simulink model "Xe_Model_Redo_June_26"  (R2018a)
settings: Solver=VariableStepAuto  StartTime=0.0  StopTime=5E5+96*60*60  RelTol=1e-3
values from neighbouring files (symbols this model uses):
  A_pipe = pi*r_pipe^2    (= 0.0126676869774)    [Startup_Script.m]
  alpha_FS = 0.517E-16    (= 5.17e-17)    [Startup_Script.m]
  alpha_G_R1 = 0.334E-17    (= 3.34e-18)    [Startup_Script.m]
  alpha_G_R2 = 0.699E-17    (= 6.99e-18)    [Startup_Script.m]
  alpha_G_R3 = 0.669E-17    (= 6.69e-18)    [Startup_Script.m]
  alpha_G_R4 = 0.791E-18    (= 7.91e-19)    [Startup_Script.m]
  D_g = 2.37E-9    (= 2.37e-09)    [Startup_Script.m]
  epsilon = 0.1    [Startup_Script.m]
  eta_b = 1E-4    (= 0.0001)    [Startup_Script.m]
  eta_fs = 1.2E-4    (= 0.00012)    [Startup_Script.m]
  f_cv = 0.004    [Startup_Script.m]
  FS_Mu_A = 4340    [Startup_Script.m]
  FS_Mu_K = 0.084    [Startup_Script.m]
  FS_Mu_MSRE = 0.007027    [Startup_Script.m]
  FS_rho_A = 3.628    [Startup_Script.m]
  FS_rho_B = 0.00066    [Startup_Script.m]
  FS_rho_MSRE = 2082    [Startup_Script.m]
  gamma_i = 0.0293524    [Startup_Script.m]
  gamma_te = 0.0322482    [Startup_Script.m]
  gamma_xe = 0.00257324    [Startup_Script.m]
  h_fc = 1.6    [Startup_Script.m]
  H_Xe_a = 5.713e-13    [Startup_Script.m]
  H_Xe_b = -7.937e-10    [Startup_Script.m]
  H_Xe_c = 2.809e-07    [Startup_Script.m]
  HX_r_Tube = ((0.5-0.042)/2)*2.54E-2    (= 0.0058166)    [Startup_Script.m]
  HX_XS = HX_N_Tubes*(pi*HX_r_Tube^2)    (= 0.0168999490356)    [Startup_Script.m]
  k_b = 1.3806E-23    (= 1.3806e-23)    [Startup_Script.m]
  lambda_i = 2.9306070546251702E-5    (= 2.93060705463e-05)    [Startup_Script.m]
  lambda_te = 0.036481430555786593    (= 0.0364814305558)    [Startup_Script.m]
  lambda_xe = 2.0924e-05    [Startup_Script.m]
  N_FC_R1 = 12    [Startup_Script.m]
  N_FC_R2 = 940    [Startup_Script.m]
  N_FC_R3 = 108    [Startup_Script.m]
  N_FC_R4 = 78    [Startup_Script.m]
  P_pump = 35420    [Startup_Script.m]
  phi0 = 3.98E+17    (= 3.98e+17)    [Startup_Script.m]
  phi_G_R_1 = mean(interp1(phi_G_R,phi_G_phi, linspace(0,r_g_r1)))    [Startup_Script.m]
  phi_G_R_2 = mean(interp1(phi_G_R,phi_G_phi, linspace(r_g_r1,r_g_r2)))    [Startup_Script.m]
  phi_G_R_3 = mean(interp1(phi_G_R,phi_G_phi, linspace(r_g_r2,r_g_r3)))    [Startup_Script.m]
  phi_G_R_4 = mean(interp1(phi_G_R,phi_G_phi, linspace(r_g_r3,r_g_r4)))    [Startup_Script.m]
  Q_strpr = 0.003155    [Startup_Script.m]
  Q_tot = 0.07571    [Startup_Script.m]
  r_b = 0.000254    [Startup_Script.m]
  r_fc = 0.79e-2    (= 0.0079)    [Startup_Script.m]
  r_pipe = (5E-2*2.54)/2    (= 0.0635)    [Startup_Script.m]
  r_xe = 2.16E-10    (= 2.16e-10)    [Startup_Script.m]
  Re_CA = 25800    [Startup_Script.m]
  Re_LH = 1E4    (= 10000)    [Startup_Script.m]
  Re_UH = 1E4    (= 10000)    [Startup_Script.m]
  sig_a_xe = 1.18E-22    (= 1.18e-22)    [Startup_Script.m]
  Sig_f = 0.15    [Startup_Script.m]
  T_CA_0 = T_INLET    (= 907.594444444)    [Startup_Script.m]
  T_FP_0 = T_OUTLET    (= 935.372222222)    [Startup_Script.m]
  T_FS_R_1_0 = mean(interp1(R_fs_m,T_fs_K, linspace(0,r_g_r1)))    [Startup_Script.m]
  T_FS_R_2_0 = mean(interp1(R_fs_m,T_fs_K, linspace(r_g_r1,r_g_r2)))    [Startup_Script.m]
  T_FS_R_3_0 = mean(interp1(R_fs_m,T_fs_K, linspace(r_g_r2,r_g_r3)))    [Startup_Script.m]
  T_FS_R_4_0 = mean(interp1(R_fs_m,T_fs_K, linspace(r_g_r3,r_g_r4)))    [Startup_Script.m]
  T_G_R_1_0 = mean(interp1(R_gr_m,T_gr_K, linspace(0,r_g_r1)))    [Startup_Script.m]
  T_HX_0 = 0.5*(T_OUTLET + T_INLET)    (= 921.483333333)    [Startup_Script.m]
  T_LH_0 = T_INLET    (= 907.594444444)    [Startup_Script.m]
  T_Mes = 928.15    [Startup_Script.m]
  T_P100_0 = T_OUTLET    (= 935.372222222)    [Startup_Script.m]
  T_P101_0 = T_OUTLET    (= 935.372222222)    [Startup_Script.m]
  T_P102_0 = T_INLET    (= 907.594444444)    [Startup_Script.m]
  T_Salt_0 = 900    [Startup_Script.m]
  T_UH_0 = T_OUTLET    (= 935.372222222)    [Startup_Script.m]
  U_FC_R1 = 0.607    [Startup_Script.m]
  U_FC_R2 = 0.183    [Startup_Script.m]
  U_FC_R3 = 0.454    [Startup_Script.m]
  U_FC_R4 = 0.250    (= 0.25)    [Startup_Script.m]
  V_CA_0 = 9.7*cubed_foot_to_cubed_meter    (= 0.274673445)    [Startup_Script.m]
  V_FP_0 = (0.9+3.2)*cubed_foot_to_cubed_meter    (= 0.116099085)    [Startup_Script.m]
  V_HX_0 = 6.1*cubed_foot_to_cubed_meter    (= 0.172732785)    [Startup_Script.m]
  V_LH_0 = 10.0*cubed_foot_to_cubed_meter    (= 0.2831685)    [Startup_Script.m]
  V_P100_0 = 2.1*cubed_foot_to_cubed_meter    (= 0.059465385)    [Startup_Script.m]
  V_P101_0 = 0.8*cubed_foot_to_cubed_meter    (= 0.02265348)    [Startup_Script.m]
  V_P102_0 = 2.2*cubed_foot_to_cubed_meter    (= 0.06229707)    [Startup_Script.m]
  V_R1_0 = V_Core_FS_0 *N_FC_R1/N_FC_tot    (= 0.00753107712766)    [Startup_Script.m]
  V_R2_0 = V_Core_FS_0 *N_FC_R2/N_FC_tot    (= 0.589934375)    [Startup_Script.m]
  V_R3_0 = V_Core_FS_0 *N_FC_R3/N_FC_tot    (= 0.0677796941489)    [Startup_Script.m]
  V_R4_0 = V_Core_FS_0 *N_FC_R4/N_FC_tot    (= 0.0489520013298)    [Startup_Script.m]
  V_UH_0 = 10.5*cubed_foot_to_cubed_meter    (= 0.297326925)    [Startup_Script.m]
undefined symbols (not defined in the file or in its folder): magnitude, V_CA, V_HX, V_P2, V_P3, V_R1, V_R2, V_R3, V_R4, V_UH
libraries: simulink x4, dspindex x4, dspstat3 x4, SignalEditorBlockLib x2
(part 1 of 11)
settings Model: Creator=terry  LastModifiedBy=terry
settings DataIOCC: SaveFormat=Array
settings DebuggingCC: UnconnectedInputMsg=error  UnconnectedOutputMsg=error  UnconnectedLineMsg=error

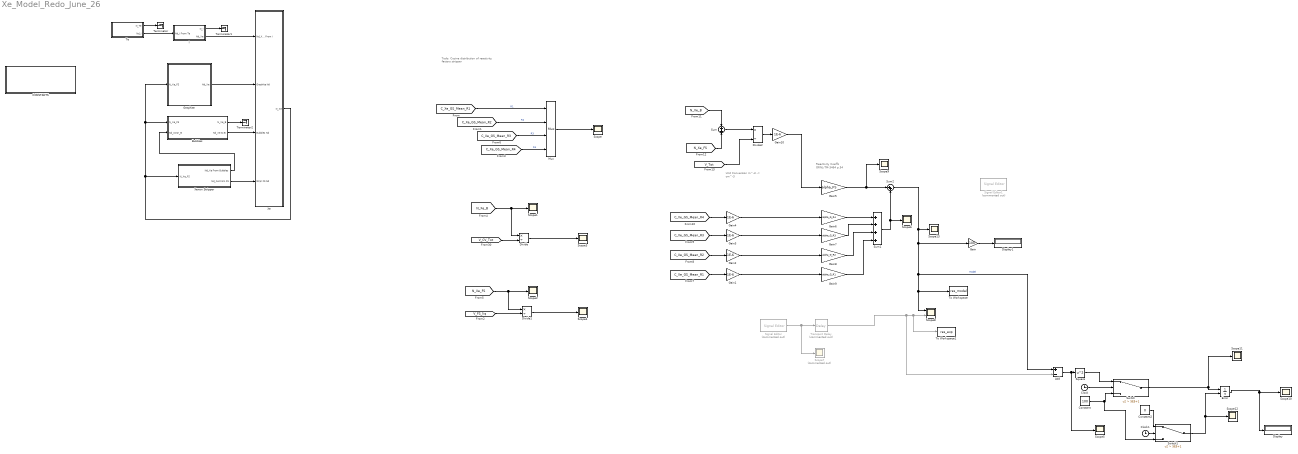
== system Xe_Model_Redo_June_26 ==
  note: Todo:
      | Cosine distribution of reactivity factors
      | stripper
  note: Reactivity Coeffs
      | ORNL-TM-3464
      | p.54
  note: Unit Conversion
      | m^-3 -> cm^-3
  Add : Sum  Inputs=+-
  Bubbles : Subsystem
  CONSTANTS : Subsystem
  Clock : Clock
  Clock1 : Clock
  Constant : Constant  Value=100
  Constant2 : Constant  Value=0
  Display : Display
  Display1 : Display
  Divide : Product  Inputs=*/
  Divide1 : Product  Inputs=*/
  Divide2 : Product  Inputs=*/
  Error : Integrator  ExternalReset=falling
  Gain : Gain  Gain=100
  Gain{1..4,10} (5 alike) : Gain  Gain=1E-6
  Gain5 : Gain  Gain=alpha_FS
  Gain6 : Gain  Gain=alpha_G_R4
  Gain7 : Gain  Gain=alpha_G_R3
  Gain8 : Gain  Gain=alpha_G_R2
  Gain9 : Gain  Gain=alpha_G_R1
  "Graphite " : Subsystem
  I : Subsystem
  Mux : Mux
  Scope{,1..6,9..13} (12 alike) : Scope
  Scope7 : Scope  Commented=on
  Scope8 : Scope  NumInputPorts=2
  Signal Editor : SignalEditorBlockLib/Signal Editor  Commented=on  FileName=MSRE_Run_10_Start_At_0_Simulink_Format.mat  ActiveScenario=exp_10  ActiveSignal=Signal  IsBus=off  OutputBusObjectStr=Bus: BusObject  SampleTime=0  Interpolate=off  ZeroCross=off  OutputAfterFinalValue=Setting to zero  Unit=inherit
  Signal Editor1 : SignalEditorBlockLib/Signal Editor  Commented=on  FileName=MSRE_Run_10_Start_At_0_Simulink_Format.mat  ActiveScenario=exp_10  ActiveSignal=Signal  IsBus=off  OutputBusObjectStr=Bus: BusObject  SampleTime=0  Interpolate=off  ZeroCross=off  OutputAfterFinalValue=Setting to zero  Unit=inherit
  Square : Math  Operator=square  SaturateOnIntegerOverflow=on
  Sum : Sum  Inputs=+|+
  Sum1 : Sum  Inputs=4
  Sum2 : Sum  Inputs=|++
  Switch : Switch  Criteria=u2 > Threshold  Threshold=5E5+1
  Switch1 : Switch  Criteria=u2 > Threshold  Threshold=5E5+1
  Te : Subsystem
  Terminator : Terminator
  Terminator1 : Terminator
  Terminator2 : Terminator
  To Workspace : ToWorkspace  VariableName=res_model  SampleTime=-1
  To Workspace1 : ToWorkspace  VariableName=res_exp  SampleTime=-1
  Transport Delay : TransportDelay  Commented=on  DelayTime=5E5
  Xe : Subsystem
  Xenon Stripper : Subsystem
  wires:
  Te/2(Nd_I) -> I/1(Nd_I From Te)
  I/2(Nd_Xe) -> Xe/1(Nd_Xe From I)
  "Graphite "/1(Nd_Xe) -> Xe/2(Graphite Nd)
  Bubbles/2(Nd_Xe to B) -> Xe/3(Bubbles Nd)
  [C_Xe_GS_Mean_R1] -> Mux/1  "R1"
  [C_Xe_GS_Mean_R2] -> Mux/2  "R2"
  [C_Xe_GS_Mean_R3] -> Mux/3  "R3"
  [C_Xe_GS_Mean_R4] -> Mux/4  "R4"
  Mux/1 -> Scope/1
  [N_Xe_B] -> Divide/1, Scope1/1
  Xe/1(N_Xe) -> "Graphite "/1(N_Xe_FS), Bubbles/1(N_Xe_FS), Xenon Stripper/1(N_Xe_FS)
  Xenon Stripper/2(Nd_Xe From FS) -> Xe/4(Strpr FS Nd)
  [V_CV_Tot] -> Divide/2
  Divide/1 -> Scope3/1
  [N_Xe_FS] -> Divide1/1, Scope2/1
  [V_FS_liq] -> Divide1/2
  Divide1/1 -> Scope4/1
  Xenon Stripper/1(Nd_Xe From Bubbles) -> Bubbles/2(Nd_strpr_B)
  [C_Xe_GS_Mean_R3] -> Gain3/1
  Sum2/1 -> Scope13/1, Add/1, Scope8/1, To Workspace/1, Gain/1  "Model"
  Sum1/1 -> Scope6/1, Sum2/2
  [C_Xe_GS_Mean_R2] -> Gain2/1
  Gain5/1 -> Scope9/1, Sum2/1
  Gain9/1 -> Sum1/4
  Signal Editor/1 -> Scope7/1, Transport Delay/1
  Gain6/1 -> Sum1/1
  Gain8/1 -> Sum1/3
  [C_Xe_GS_Mean_R1] -> Gain1/1
  Gain7/1 -> Sum1/2
  [C_Xe_GS_Mean_R4] -> Gain4/1
  [N_Xe_FS] -> Sum/2
  [N_Xe_B] -> Sum/1
  Sum/1 -> Divide2/1
  [V_Tot] -> Divide2/2
  Divide2/1 -> Gain10/1
  Clock/1 -> Switch/2
  Transport Delay/1 -> Add/2, To Workspace1/1, Scope8/2
  Add/1 -> Scope5/1, Square/1
  Error/1 -> Display/1, Scope10/1
  Switch/1 -> Error/1, Scope11/1
  Constant/1 -> Switch1/3, Switch/3
  Clock1/1 -> Switch1/2
  Constant2/1 -> Switch1/1
  Switch1/1 -> Scope12/1, Error/2
  Square/1 -> Switch/1
  Gain4/1 -> Gain6/1
  Gain3/1 -> Gain7/1
  Gain2/1 -> Gain8/1
  Gain1/1 -> Gain9/1
  Gain10/1 -> Gain5/1
  Te/1(N_Te) -> Terminator/1
  I/1(N_I) -> Terminator1/1
  Bubbles/1(N_Xe_B) -> Terminator2/1
  Gain/1 -> Display1/1

== system Xe_Model_Redo_June_26/Bubbles ==
  note: Fix Stripper
  note: Positive Values of Nd_Xe to B are going TO the bubbles
  N_Xe_FS : Inport
  Nd_strpr_B : Inport  Port=2
  Bubble Mass Transfer : Subsystem
  Burnout : Subsystem
  Integrator : Integrator
  Sum : Sum  Inputs=+---
  Xe Decay : Subsystem
  N_Xe_B : Outport
  Nd_Xe to B : Outport  Port=2
  tag scope: N_Xe_B=global
  wires:
  Sum/1 -> Integrator/1
  Integrator/1 -> N_Xe_B/1, Burnout/1(N_Xe_B), Bubble Mass Transfer/2(N_Xe_B), Xe Decay/1(N_Xe_B), [N_Xe_B]  "N_Xe_B"
  N_Xe_FS/1 -> Bubble Mass Transfer/1(N_Xe_FS)
  Bubble Mass Transfer/1(Nd_Xe) -> Nd_Xe to B/1, Sum/1
  Burnout/1(Nd_Xe) -> Sum/2
  Xe Decay/1(Nd_Xe) -> Sum/3
  Nd_strpr_B/1 -> Sum/4

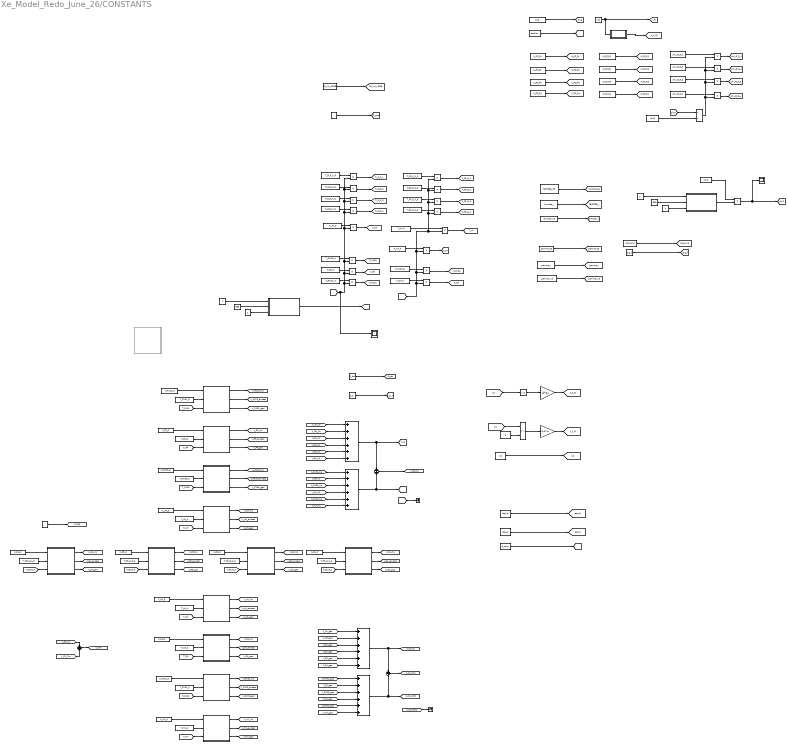
== system Xe_Model_Redo_June_26/CONSTANTS ==
  note: Total Volume
  note: Stripper
  note: Pipe Radius
  note: Flow Rate
  note: Area of 1 Bubble
  note: Bubble
  note: CV Gas Vol.
  note: Liq FS Vol.
  note: CV Fraction
  note: HX
  note: Graphite
  note: Scale by the %FP
  note: Graphite N0 Flux
  note: Constants
  note: Number of FC
  note: Material Properties
  note: Channel Salt Velocity
  note: Graphite
  note: Volumes
  note: X-SECTION DATA
  note: Neutron Flux
  note: Nuclear Data
  note: Decay Constants
  note: Fission Yields (From U235)
  note: 1/m
  note: Got this from Serpent Model
  note: Surface
      | Area of one
      | Fuel Channel
  note: Themal
  note: Graphite
  note: Volume of 1 Bubble
  Constant : Constant  Value=phi0
  Constant1 : Constant  Value=lambda_xe
  Constant10 : Constant  Value=Sig_f
  Constant11 : Constant  Value=epsilon
  Constant12 : Constant  Value=U_FC_R2
  Constant13 : Constant  Value=U_FC_R3
  Constant14 : Constant  Value=U_FC_R4  VectorParams1D=off
  Constant15 : Constant  Value=r_fc
  Constant16 : Constant  Value=N_FC_R2
  Constant17 : Constant  Value=V_R1_0
  Constant{18,44..45,79} (4 alike) : Constant
  Constant19 : Constant  Value=V_R2_0
  Constant2 : Constant  Value=FS_Mu_MSRE
  Constant20 : Constant  Value=8.314
  Constant21 : Constant  Value=phi_G_R_2
  Constant22 : Constant  Value=phi_G_R_1
  Constant23 : Constant  Value=phi_G_R_3
  Constant24 : Constant  Value=phi_G_R_4
  Constant25 : Constant  Value=N_FC_R1
  Constant26 : Constant  Value=U_FC_R1
  Constant27 : Constant  Value=N_FC_R3
  Constant28 : Constant  Value=N_FC_R4
  Constant29 : Constant  Value=phi0
  Constant3 : Constant  Value=f_cv
  Constant30 : Constant  Value=T_HX_0  OutDataTypeStr=Inherit: Inherit via back propagation
  Constant{31..33,38} (4 alike) : Constant  Value=T_G_R_1_0
  Constant{34..35,37,39,50} (5 alike) : Constant  Value=T_FS_R_1_0
  Constant36 : Constant  Value=5E5
  Constant4 : Constant  Value=sig_a_xe
  Constant40 : Constant  Value=T_P100_0
  Constant41 : Constant  Value=T_FP_0
  Constant42 : Constant  Value=T_P101_0
  Constant43 : Constant  Value=T_UH_0
  Constant46 : Constant  Value=T_CA_0
  Constant47 : Constant  Value=T_FS_R_2_0
  Constant48 : Constant  Value=T_LH_0
  Constant49 : Constant  Value=T_P102_0
  Constant5 : Constant  Value=lambda_i
  Constant51 : Constant  Value=V_R3_0
  Constant52 : Constant  Value=T_FS_R_3_0
  Constant53 : Constant  Value=V_R4_0
  Constant54 : Constant  Value=T_FS_R_4_0
  Constant55 : Constant  Value=V_CA_0
  Constant56 : Constant  Value=T_CA_0
  Constant57 : Constant  Value=V_P102_0
  Constant58 : Constant  Value=T_P102_0
  Constant59 : Constant  Value=V_LH_0
  Constant6 : Constant  Value=lambda_te
  Constant60 : Constant  Value=T_LH_0
  Constant61 : Constant  Value=V_HX_0
  Constant62 : Constant  Value=T_HX_0
  Constant63 : Constant  Value=V_UH_0
  Constant64 : Constant  Value=T_UH_0
  Constant65 : Constant  Value=V_P100_0
  Constant66 : Constant  Value=T_P100_0
  Constant67 : Constant  Value=V_FP_0
  Constant68 : Constant  Value=T_FP_0
  Constant69 : Constant  Value=V_P101_0
  Constant7 : Constant  Value=gamma_xe
  Constant70 : Constant  Value=T_P101_0
  Constant71 : Constant  Value=3
  Constant72 : Constant  Value=Q_tot
  Constant73 : Constant  Value=r_b
  Constant74 : Constant  Value=r_pipe
  Constant75 : Constant  Value=eta_fs
  Constant76 : Constant  Value=eta_b
  Constant77 : Constant  Value=Q_strpr
  Constant78 : Constant  Value=5E5
  Constant8 : Constant  Value=gamma_i
  Constant9 : Constant  Value=gamma_te
  D_g : Constant  Value=D_g
  Divide1 : Product  Inputs=*/
  Fuel Channel Area : Subsystem
  Gain : Gain  Gain=4*pi
  Gain1 : Gain  Gain=(4/3)*pi
  Math Function : Math  Operator=pow  SaturateOnIntegerOverflow=on
  Multiply{,1..19} (20 alike) : Product
  Product12 : Product
  Scope : Scope
  Scope1 : Scope
  Square : Math  Operator=square  SaturateOnIntegerOverflow=on
  Subsystem : Subsystem
  Subsystem1 : Subsystem
  Sum{,1,3..4} (4 alike) : Sum  Inputs=++++++
  Sum2 : Sum  Inputs=+|+
  Sum5 : Sum  Inputs=+|+
  Sum6 : Sum  Inputs=+|+
  Terminator : Terminator
  Terminator1 : Terminator
  V CA : Subsystem
  V FP : Subsystem
  V FP1 : Subsystem  Commented=on
  V HX : Subsystem
  V LH : Subsystem
  V P100 : Subsystem
  V P101 : Subsystem
  V P102 : Subsystem
  V R1 : Subsystem
  V R2 : Subsystem
  V R3 : Subsystem
  V R4 : Subsystem
  V UH : Subsystem
  tag scope: A_1_B=global, A_1_FC=global, D_g=global, FS_Mu_MSRE=global, N_FC_R1=global, N_FC_R2=global, N_FC_R3=global, N_FC_R4=global, Q_strpr=global, Q_tot=global, R_gas=global, Sig_f=global, T_CA=global, T_FP=global, T_FS_R_1=global, T_FS_R_2=global, T_FS_R_3=global, T_FS_R_4=global, T_G_R_1=global, T_G_R_2=global, T_G_R_3=global, T_G_R_4=global, T_HX=global, T_LH=global, T_P100=global, T_P101=global, T_P102=global, T_UH=global, U_FC_R1=global, U_FC_R2=global, U_FC_R3=global, U_FC_R4=global, V_1_B=global, V_CA_excess=global, V_CA_gas=global, V_CA_liq=global, V_CV_IC=global, V_CV_OOC=global, V_CV_Tot=global, V_FP_excess=global, V_FP_gas=global, V_FP_liq=global, V_FS_liq=global, V_HX_excess=global, V_HX_gas=global, V_HX_liq=global, V_IC=global, V_LH_excess=global, V_LH_gas=global, V_LH_liq=global, V_OOC=global, V_P100_excess=global, V_P100_gas=global, V_P100_liq=global, V_P101_excess=global, V_P101_gas=global, V_P101_liq=global, V_P102_excess=global, V_P102_gas=global, V_P102_liq=global, V_R1_excess=global, V_R1_gas=global, V_R1_liq=global, V_R2_excess=global, V_R2_gas=global, V_R2_liq=global, V_R3_excess=global, V_R3_gas=global, V_R3_liq=global, V_R4_excess=global, V_R4_gas=global, V_R4_liq=global, V_Tot=global, V_UH_excess=global, V_UH_gas=global, V_UH_liq=global, epsilon=global, eta_b=global, eta_fs=global, f_cv_0=global, gamma_i=global, gamma_te=global, gamma_xe=global, lambda_i=global, lambda_te=global, lambda_xe=global, phi0=global, phi_G_R_1=global, phi_G_R_2=global, phi_G_R_3=global, phi_G_R_4=global, r_b=global, r_fc=global, r_pipe=global, sig_a_xe=global
  wires:
  Constant36/1 -> Subsystem/2(Switch Time)
  Constant18/1 -> Subsystem/1(After Val)  "Drop"
  Subsystem/1(Out) -> Product12/2
  Constant45/1 -> Subsystem/3(Before Val)
  Constant6/1 -> [lambda_te]
  Constant1/1 -> [lambda_xe]
  Constant5/1 -> [lambda_i]
  D_g/1 -> [D_g]
  Constant11/1 -> [epsilon]
  Constant12/1 -> [U_FC_R2]
  Constant13/1 -> [U_FC_R3]
  Constant14/1 -> [U_FC_R4]
  Constant26/1 -> [U_FC_R1]
  Constant15/1 -> Fuel Channel Area/1(r), [r_fc]
  Fuel Channel Area/1(A_1_fc) -> [A_1_FC]
  Constant28/1 -> [N_FC_R4]
  Constant16/1 -> [N_FC_R2]
  Constant27/1 -> [N_FC_R3]
  Constant25/1 -> [N_FC_R1]
  Constant20/1 -> [R_gas]
  [phi0] -> Divide1/1
  Multiply/1 -> [phi_G_R_4]
  Divide1/1 -> Multiply/2, Multiply1/2, Multiply2/2, Multiply3/2
  Multiply1/1 -> [phi_G_R_3]
  Multiply2/1 -> [phi_G_R_2]
  Multiply3/1 -> [phi_G_R_1]
  Constant50/1 -> V R1/2(T_0)
  [T_FS_R_1] -> V R1/3(T)
  V R1/2(V_excess_liq) -> [V_R1_excess]
  V R1/3(V_gas) -> [V_R1_gas]
  V R1/1(V_liq) -> [V_R1_liq]
  Constant47/1 -> V R2/2(T_0)
  V R2/1(V_liq) -> [V_R2_liq]
  V R2/2(V_excess_liq) -> [V_R2_excess]
  V R2/3(V_gas) -> [V_R2_gas]
  [T_FS_R_2] -> V R2/3(T)
  Constant52/1 -> V R3/2(T_0)
  V R3/1(V_liq) -> [V_R3_liq]
  V R3/2(V_excess_liq) -> [V_R3_excess]
  V R3/3(V_gas) -> [V_R3_gas]
  [T_FS_R_3] -> V R3/3(T)
  Constant54/1 -> V R4/2(T_0)
  V R4/1(V_liq) -> [V_R4_liq]
  V R4/2(V_excess_liq) -> [V_R4_excess]
  V R4/3(V_gas) -> [V_R4_gas]
  [T_FS_R_4] -> V R4/3(T)
  Constant56/1 -> V CA/2(T_0)
  V CA/3(V_gas) -> [V_CA_gas]
  [T_CA] -> V CA/3(T)
  V CA/1(V_liq) -> [V_CA_liq]
  V CA/2(V_excess_liq) -> [V_CA_excess]
  V P102/1(V_liq) -> [V_P102_liq]
  V P102/2(V_excess_liq) -> [V_P102_excess]
  [T_P102] -> V P102/3(T)
  V P102/3(V_gas) -> [V_P102_gas]
  Constant58/1 -> V P102/2(T_0)
  V LH/1(V_liq) -> [V_LH_liq]
  V LH/2(V_excess_liq) -> [V_LH_excess]
  [T_LH] -> V LH/3(T)
  V LH/3(V_gas) -> [V_LH_gas]
  Constant60/1 -> V LH/2(T_0)
  Constant62/1 -> V HX/2(T_0)
  [T_HX] -> V HX/3(T)
  V HX/2(V_excess_liq) -> [V_HX_excess]
  V HX/1(V_liq) -> [V_HX_liq]
  V HX/3(V_gas) -> [V_HX_gas]
  V UH/3(V_gas) -> [V_UH_gas]
  [T_UH] -> V UH/3(T)
  V UH/2(V_excess_liq) -> [V_UH_excess]
  Constant64/1 -> V UH/2(T_0)
  V UH/1(V_liq) -> [V_UH_liq]
  Constant66/1 -> V P100/2(T_0)
  [T_P100] -> V P100/3(T)
  V P100/2(V_excess_liq) -> [V_P100_excess]
  V P100/1(V_liq) -> [V_P100_liq]
  V P100/3(V_gas) -> [V_P100_gas]
  V FP/2(FP Excess) -> [V_FP_excess]
  Constant68/1 -> V FP/2(T_0)
  [T_FP] -> V FP/3(T)
  [T_P101] -> V P101/3(T)
  V P101/2(V_excess_liq) -> [V_P101_excess]
  Constant70/1 -> V P101/2(T_0)
  [V_UH_liq] -> Sum/2
  [V_R1_liq] -> Sum/3
  [V_R2_liq] -> Sum/4
  [V_R3_liq] -> Sum/5
  [V_R4_liq] -> Sum/6
  [V_P101_liq] -> Sum1/1
  [V_FP_liq] -> Sum1/2
  [V_CA_liq] -> Sum1/4
  [V_P102_liq] -> Sum1/5
  [V_HX_liq] -> Sum1/6
  Sum1/1 -> Sum2/2, [V_OOC]
  Sum2/1 -> [V_FS_liq]
  Sum/1 -> [V_IC], Sum2/1
  [V_P100_liq] -> Sum1/3
  [V_LH_liq] -> Sum/1
  [V_R2_gas] -> Sum3/4
  [V_UH_gas] -> Sum3/2
  [V_P101_gas] -> Sum4/1
  [V_CA_gas] -> Sum4/4
  [V_HX_gas] -> Sum4/6
  Sum3/1 -> [V_CV_IC], Sum5/1
  [V_P100_gas] -> Sum4/3
  [V_R4_gas] -> Sum3/6
  Sum5/1 -> [V_CV_Tot]
  [V_R1_gas] -> Sum3/3
  [V_R3_gas] -> Sum3/5
  [V_FP_gas] -> Sum4/2
  Sum4/1 -> [V_CV_OOC], Sum5/2
  [V_LH_gas] -> Sum3/1
  [V_P102_gas] -> Sum4/5
  [r_b] -> Square/1
  Square/1 -> Gain/1
  Gain/1 -> [A_1_B]
  Math Function/1 -> Gain1/1
  Gain1/1 -> [V_1_B]
  [r_b] -> Math Function/1
  Constant71/1 -> Math Function/2
  Constant72/1 -> [Q_tot]
  Constant74/1 -> [r_pipe]
  [V_FS_liq] -> Sum6/1
  [V_CV_Tot] -> Sum6/2
  Sum6/1 -> [V_Tot]
  V P101/1(V_liq) -> [V_P101_liq]
  V P101/3(V_gas) -> [V_P101_gas]
  V FP/1(V_liq) -> [V_FP_liq]
  V FP/3(V_gas) -> [V_FP_gas]
  Product12/1 -> [phi0], Scope/1
  Constant53/1 -> V R4/1(V_0)
  Constant51/1 -> V R3/1(V_0)
  Constant19/1 -> V R2/1(V_0)
  Constant17/1 -> V R1/1(V_0)
  Constant63/1 -> V UH/1(V_0)
  Constant59/1 -> V LH/1(V_0)
  Constant69/1 -> V P101/1(V_0)
  Constant67/1 -> V FP/1(V_0)
  Constant65/1 -> V P100/1(V_0)
  Constant55/1 -> V CA/1(V_0)
  Constant57/1 -> V P102/1(V_0)
  Constant61/1 -> V HX/1(V_0)
  Constant9/1 -> [gamma_te]
  Constant8/1 -> [gamma_i]
  Constant7/1 -> [gamma_xe]
  Constant10/1 -> [Sig_f]
  Constant4/1 -> [sig_a_xe]
  Constant29/1 -> Divide1/2
  Constant/1 -> Product12/1
  Constant24/1 -> Multiply/1
  Constant23/1 -> Multiply1/1
  Constant21/1 -> Multiply2/1
  Constant22/1 -> Multiply3/1
  Constant76/1 -> [eta_b]
  Constant75/1 -> [eta_fs]
  Constant77/1 -> [Q_strpr]
  Constant73/1 -> [r_b]
  Constant3/1 -> [f_cv_0]
  Constant2/1 -> [FS_Mu_MSRE]
  [V_OOC] -> Terminator/1
  [V_CV_OOC] -> Terminator1/1
  Constant38/1 -> Multiply4/1
  Constant31/1 -> Multiply5/1
  Constant32/1 -> Multiply6/1
  Constant33/1 -> Multiply7/1
  Constant43/1 -> Multiply8/1
  Constant40/1 -> Multiply9/1
  Constant41/1 -> Multiply10/1
  Constant42/1 -> Multiply11/1
  Constant39/1 -> Multiply12/1
  Constant34/1 -> Multiply13/1
  Constant35/1 -> Multiply14/1
  Constant37/1 -> Multiply15/1
  Constant48/1 -> Multiply16/1
  Constant30/1 -> Multiply17/1
  Constant49/1 -> Multiply18/1
  Constant46/1 -> Multiply19/1
  Multiply18/1 -> [T_P102]
  Multiply19/1 -> [T_CA]
  Multiply17/1 -> [T_HX]
  Multiply16/1 -> [T_LH]
  Multiply15/1 -> [T_FS_R_4]
  Multiply14/1 -> [T_FS_R_3]
  Multiply13/1 -> [T_FS_R_2]
  Multiply12/1 -> [T_FS_R_1]
  Multiply4/1 -> [T_G_R_1]
  Multiply5/1 -> [T_G_R_2]
  Multiply6/1 -> [T_G_R_3]
  Multiply7/1 -> [T_G_R_4]
  Multiply8/1 -> [T_UH]
  Multiply9/1 -> [T_P100]
  Multiply10/1 -> [T_FP]
  Multiply11/1 -> [T_P101]
  [T_Gain] -> Scope1/1, Multiply7/2, Multiply6/2, Multiply4/2, Multiply5/2, Multiply8/2, Multiply9/2, Multiply10/2, Multiply11/2
  [T_Gain] -> Multiply18/2, Multiply12/2, Multiply13/2, Multiply14/2, Multiply15/2, Multiply16/2, Multiply17/2, Multiply19/2
  Constant44/1 -> Subsystem1/1(After Val)  "Drop"
  Constant79/1 -> Subsystem1/3(Before Val)
  Constant78/1 -> Subsystem1/2(Switch Time)
  Subsystem1/1(Out) -> [T_Gain]

== system Xe_Model_Redo_June_26/Graphite  ==
  N_Xe_FS : Inport
  Graphite Region 1 : Subsystem
  Graphite Region 2 : Subsystem
  Graphite Region 3 : Subsystem
  Graphite Region 4 : Subsystem
  Sum : Sum  Inputs=++++
  Terminator{,1..3} (4 alike) : Terminator
  Nd_Xe : Outport
  tag scope: C_Xe_GS_Mean_R1=global, C_Xe_GS_Mean_R2=global, C_Xe_GS_Mean_R3=global, C_Xe_GS_Mean_R4=global
  wires:
  N_Xe_FS/1 -> Graphite Region 4/1(N_Xe_FS), Graphite Region 3/1(N_Xe_FS), Graphite Region 2/1(N_Xe_FS), Graphite Region 1/1(N_Xe_FS)
  Graphite Region 1/3(Nd_Xe_FS->GS) -> Sum/1
  Graphite Region 3/3(Nd_Xe_FS->GS) -> Sum/3
  Graphite Region 4/3(Nd_Xe_FS->GS) -> Sum/4
  Graphite Region 4/2(C_Xe_GS_Mean) -> [C_Xe_GS_Mean_R4]
  Graphite Region 1/2(C_Xe_GS_Mean) -> [C_Xe_GS_Mean_R1]
  Graphite Region 2/3(Nd_Xe_FS->GS) -> Sum/2
  Sum/1 -> Nd_Xe/1
  Graphite Region 2/2(C_Xe_GS_Mean) -> [C_Xe_GS_Mean_R2]
  Graphite Region 3/2(C_Xe_GS_Mean) -> [C_Xe_GS_Mean_R3]
  Graphite Region 1/1(C_Xe_GS_Max) -> Terminator/1
  Graphite Region 2/1(C_Xe_GS_Max) -> Terminator1/1
  Graphite Region 3/1(C_Xe_GS_Max) -> Terminator2/1
  Graphite Region 4/1(C_Xe_GS_Max) -> Terminator3/1

== system Xe_Model_Redo_June_26/I ==
  Nd_I From Te : Inport
  Display1 : Display
      settings: Format=short_e
  I Decay : Subsystem
  I From Fission : Subsystem
  Integrator : Integrator
  Scope : Scope
  Sum : Sum  Inputs=++-
  N_I : Outport
  Nd_Xe : Outport  Port=2
  wires:
  Integrator/1 -> Scope/1, N_I/1, I Decay/1(N_I)  "N_I"
  Sum/1 -> Integrator/1
  I Decay/1(Nd_I) -> Sum/3, Nd_Xe/1
  Nd_I From Te/1 -> Sum/1, Display1/1
  I From Fission/1(Nd_I) -> Sum/2

== system Xe_Model_Redo_June_26/Te ==
  Integrator : Integrator
  Sum : Sum  Inputs=|+-
  Te Decay : Subsystem
  Te From Fission : Subsystem
  N_Te : Outport
  Nd_I : Outport  Port=2
  wires:
  Integrator/1 -> N_Te/1, Te Decay/1(n_te)  "n_te"
  Te Decay/1(nd_te) -> Nd_I/1, Sum/2
  Sum/1 -> Integrator/1
  Te From Fission/1(nd_te) -> Sum/1

== system Xe_Model_Redo_June_26/Xe ==
  Nd_Xe From I : Inport
  Graphite Nd : Inport  Port=2
  Bubbles Nd : Inport  Port=3
  Strpr FS Nd : Inport  Port=4
  Burnout : Subsystem
  Integrator : Integrator
  Scope : Scope
  Scope1 : Scope
  Scope2 : Scope
  Sum : Sum  Inputs=++-----
      mask Display:
      | port_label('input', 1, '+ From I')
      | port_label('input', 2, '+ From Fiss.')
      | port_label('input', 3, '- From Decay')
      | port_label('input', 4, '- From Burnout')
      | port_label('input', 5, '- From Graphite MT')
      | port_label('input', 6, '- From Bubble MT')
      | port_label('input', 7, '- From Strpr (FS)')
  Xe Decay : Subsystem
  Xe From Fission : Subsystem
  N_Xe : Outport
  tag scope: N_Xe_FS=global
  wires:
  Integrator/1 -> N_Xe/1, Scope/1, Burnout/1(N_Xe), Xe Decay/1(N_Xe), [N_Xe_FS]  "N_Xe"
  Sum/1 -> Integrator/1
  Xe Decay/1(Nd_Xe) -> Sum/3
  Nd_Xe From I/1 -> Sum/1
  Graphite Nd/1 -> Sum/5
  Bubbles Nd/1 -> Sum/6
  Strpr FS Nd/1 -> Sum/7
  Burnout/1(Nd_Xe) -> Scope2/1, Sum/4
  Xe From Fission/1(Nd_Xe) -> Scope1/1, Sum/2

== system Xe_Model_Redo_June_26/Xenon Stripper ==
  N_Xe_FS : Inport
  Bubble Stripping : Subsystem
  Fuel Salt Concentration atoms/m^3 : Subsystem
  Fuel Salt Stripping : Subsystem
  Nd_Xe From Bubbles : Outport
  Nd_Xe From FS : Outport  Port=2
  wires:
  [Q_strpr] -> Bubble Stripping/1(Stripper Flowrate [m^3/sec]), Fuel Salt Stripping/1(Stripper Fowrate [m^3/sec])
  N_Xe_FS/1 -> Fuel Salt Concentration atoms/m^3/1(N_FS)
  Bubble Stripping/1(Removal of xenon from bubbles) -> Nd_Xe From Bubbles/1
  Fuel Salt Concentration atoms/m^3/1(C_FS) -> Fuel Salt Stripping/2(Fuel Salt Concentration [atoms/m^3])
  Fuel Salt Stripping/1(Fuel Salt Remvoal rate [atoms/sec]) -> Nd_Xe From FS/1

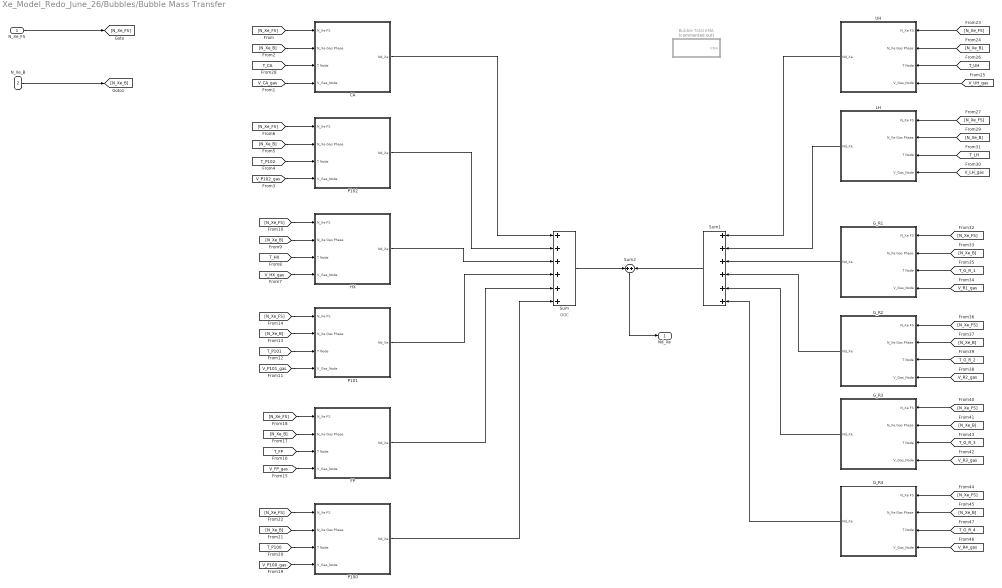
== system Xe_Model_Redo_June_26/Bubbles/Bubble Mass Transfer ==
  note: OOC
  N_Xe_FS : Inport
  N_Xe_B : Inport  Port=2
  Bubble Total KMA : Subsystem  Commented=on
  CA : Subsystem
  FP : Subsystem
  G_R1 : Subsystem
  G_R2 : Subsystem
  G_R3 : Subsystem
  G_R4 : Subsystem
  HX : Subsystem
  LH : Subsystem
  P100 : Subsystem
  P101 : Subsystem
  P102 : Subsystem
  Sum : Sum  Inputs=6
  Sum1 : Sum  Inputs=6
  Sum2 : Sum  Inputs=+|+
  UH : Subsystem
  Nd_Xe : Outport
  wires:
  [T_CA] -> CA/3(T Node)
  [V_CA_gas] -> CA/4(V_Gas_Node)
  N_Xe_FS/1 -> [N_Xe_FS]
  N_Xe_B/1 -> [N_Xe_B]
  [N_Xe_FS] -> CA/1(N_Xe FS)
  [N_Xe_B] -> CA/2(N_Xe Gas Phase)
  [V_P102_gas] -> P102/4(V_Gas_Node)
  [T_P102] -> P102/3(T Node)
  [N_Xe_B] -> P102/2(N_Xe Gas Phase)
  [N_Xe_FS] -> P102/1(N_Xe FS)
  CA/1(Nd_Xe) -> Sum/1
  P102/1(Nd_Xe) -> Sum/2
  HX/1(Nd_Xe) -> Sum/3
  FP/1(Nd_Xe) -> Sum/5
  P100/1(Nd_Xe) -> Sum/6
  [V_HX_gas] -> HX/4(V_Gas_Node)
  [T_HX] -> HX/3(T Node)
  [N_Xe_B] -> HX/2(N_Xe Gas Phase)
  [N_Xe_FS] -> HX/1(N_Xe FS)
  [N_Xe_FS] -> P101/1(N_Xe FS)
  [N_Xe_B] -> P101/2(N_Xe Gas Phase)
  [V_P101_gas] -> P101/4(V_Gas_Node)
  [T_P101] -> P101/3(T Node)
  [N_Xe_FS] -> FP/1(N_Xe FS)
  [N_Xe_B] -> FP/2(N_Xe Gas Phase)
  [V_FP_gas] -> FP/4(V_Gas_Node)
  [T_FP] -> FP/3(T Node)
  [N_Xe_FS] -> P100/1(N_Xe FS)
  [N_Xe_B] -> P100/2(N_Xe Gas Phase)
  [V_P100_gas] -> P100/4(V_Gas_Node)
  [T_P100] -> P100/3(T Node)
  G_R1/1(Nd_Xe) -> Sum1/3
  G_R4/1(Nd_Xe) -> Sum1/6
  UH/1(Nd_Xe) -> Sum1/1
  [N_Xe_FS] -> UH/1(N_Xe FS)
  [N_Xe_B] -> UH/2(N_Xe Gas Phase)
  [T_UH] -> UH/3(T Node)
  [V_UH_gas] -> UH/4(V_Gas_Node)
  Sum/1 -> Sum2/1
  Sum1/1 -> Sum2/2
  [V_LH_gas] -> LH/4(V_Gas_Node)
  [N_Xe_B] -> LH/2(N_Xe Gas Phase)
  [N_Xe_FS] -> LH/1(N_Xe FS)
  [T_LH] -> LH/3(T Node)
  LH/1(Nd_Xe) -> Sum1/2
  [T_G_R_1] -> G_R1/3(T Node)
  [N_Xe_B] -> G_R1/2(N_Xe Gas Phase)
  [V_R1_gas] -> G_R1/4(V_Gas_Node)
  [N_Xe_FS] -> G_R1/1(N_Xe FS)
  [V_R2_gas] -> G_R2/4(V_Gas_Node)
  [T_G_R_2] -> G_R2/3(T Node)
  [N_Xe_B] -> G_R2/2(N_Xe Gas Phase)
  [N_Xe_FS] -> G_R2/1(N_Xe FS)
  G_R2/1(Nd_Xe) -> Sum1/4
  [V_R3_gas] -> G_R3/4(V_Gas_Node)
  [T_G_R_3] -> G_R3/3(T Node)
  [N_Xe_B] -> G_R3/2(N_Xe Gas Phase)
  [N_Xe_FS] -> G_R3/1(N_Xe FS)
  G_R3/1(Nd_Xe) -> Sum1/5
  [V_R4_gas] -> G_R4/4(V_Gas_Node)
  [T_G_R_4] -> G_R4/3(T Node)
  [N_Xe_B] -> G_R4/2(N_Xe Gas Phase)
  [N_Xe_FS] -> G_R4/1(N_Xe FS)
  Sum2/1 -> Nd_Xe/1
  P101/1(Nd_Xe) -> Sum/4

== system Xe_Model_Redo_June_26/Bubbles/Burnout ==
  note: Concentration in all of gas phase
  note: Burnout only occurs in core. We only care about the gas phase burnout here.
  N_Xe_B : Inport
  Divide : Product  Inputs=*/
  Product : Product  Inputs=4
  Nd_Xe : Outport
  wires:
  [phi0] -> Product/2
  [sig_a_xe] -> Product/3
  Product/1 -> Nd_Xe/1
  Divide/1 -> Product/1
  N_Xe_B/1 -> Divide/1
  [V_CV_Tot] -> Divide/2
  [V_CV_IC] -> Product/4

== system Xe_Model_Redo_June_26/Bubbles/Xe Decay ==
  N_Xe_B : Inport
  Product : Product
  Nd_Xe : Outport
  wires:
  Product/1 -> Nd_Xe/1
  [lambda_xe] -> Product/2
  N_Xe_B/1 -> Product/1

== system Xe_Model_Redo_June_26/CONSTANTS/Fuel Channel Area ==
  r : Inport
  Constant : Constant  Value=h_fc
  Constant23 : Constant  Value=2*pi
  Product1 : Product  Inputs=3
  A_1_fc : Outport
  wires:
  r/1 -> Product1/1
  Product1/1 -> A_1_fc/1
  Constant23/1 -> Product1/2
  Constant/1 -> Product1/3

== system Xe_Model_Redo_June_26/CONSTANTS/Subsystem ==
  After Val : Inport
  Switch Time : Inport  Port=2
  Before Val : Inport  Port=3
  Clock : Clock
  Subtract : Sum  Inputs=+-
  Switch : Switch  Criteria=u2 > Threshold
  Out : Outport
  wires:
  Subtract/1 -> Switch/2
  Switch Time/1 -> Subtract/2
  After Val/1 -> Switch/1
  Clock/1 -> Subtract/1
  Before Val/1 -> Switch/3
  Switch/1 -> Out/1

== system Xe_Model_Redo_June_26/CONSTANTS/Subsystem1 ==
  After Val : Inport
  Switch Time : Inport  Port=2
  Before Val : Inport  Port=3
  Clock : Clock
  Subtract : Sum  Inputs=+-
  Switch : Switch  Criteria=u2 > Threshold
  Out : Outport
  wires:
  Subtract/1 -> Switch/2
  Switch Time/1 -> Subtract/2
  After Val/1 -> Switch/1
  Clock/1 -> Subtract/1
  Before Val/1 -> Switch/3
  Switch/1 -> Out/1

== system Xe_Model_Redo_June_26/CONSTANTS/V CA ==
  note: Total Current Vol
  note: FS Volume W Thermal Expansion
  V_0 : Inport
  T_0 : Inport  Port=2
  T : Inport  Port=3
  Current Density : Subsystem
  Current volume (liq) : Product  Inputs=*/
  Display : Display
      settings: Format=short_e
  Gain Gain : Subsystem
  Nominal Mass of Fuel Salt : Product
  Nominal gas volume : Product
  Nominal liquid volume : Sum  Inputs=+-
  Reference Density : Subsystem
  Subtract : Sum  Inputs=-+
  Sum : Sum
  Sum1 : Sum  Inputs=+-
  V_liq : Outport
  V_excess_liq : Outport  Port=2
  V_gas : Outport  Port=3
  wires:
  Nominal Mass of Fuel Salt/1 -> Current volume (liq)/1
  Current Density/1(rho_FS [kg/m^3]) -> Current volume (liq)/2
  Nominal liquid volume/1 -> Nominal Mass of Fuel Salt/1
  Reference Density/1(rho_FS [kg/m^3]) -> Nominal Mass of Fuel Salt/2
  V_0/1 -> Display/1, Sum1/1, Subtract/1, Nominal liquid volume/1, Nominal gas volume/1
  Current volume (liq)/1 -> Sum/1
  T_0/1 -> Gain Gain/3("T_0 "), Reference Density/1(T_Salt [k])
  Subtract/1 -> V_excess_liq/1
  [f_cv_0] -> Nominal gas volume/2
  Nominal gas volume/1 -> Gain Gain/1(Vol. Gas 0), Nominal liquid volume/2
  T/1 -> Gain Gain/2(T), Current Density/1(T_Salt [k])
  Sum/1 -> Subtract/2
  Gain Gain/1(V Gas) -> V_gas/1, Sum1/2, Sum/2
  Sum1/1 -> V_liq/1

== system Xe_Model_Redo_June_26/CONSTANTS/V FP ==
  note: Total Current Vol
  note: FS Volume W Thermal Expansion
  V_0 : Inport
  T_0 : Inport  Port=2
  T : Inport  Port=3
  Current Density : Subsystem
  Current volume (liq) : Product  Inputs=*/
  Display : Display
      settings: Format=short_e
  Gain Gain : Subsystem
  Nominal Mass of Fuel Salt : Product
  Nominal gas volume : Product
  Nominal liquid volume : Sum  Inputs=+-
  Reference Density : Subsystem
  Subtract : Sum  Inputs=-+
  Sum : Sum
  Sum3 : Sum  Inputs=12
  V_liq : Outport
  FP Excess : Outport  Port=2
  V_gas : Outport  Port=3
  wires:
  Nominal Mass of Fuel Salt/1 -> Current volume (liq)/1
  Current Density/1(rho_FS [kg/m^3]) -> Current volume (liq)/2
  Nominal liquid volume/1 -> Nominal Mass of Fuel Salt/1
  Reference Density/1(rho_FS [kg/m^3]) -> Nominal Mass of Fuel Salt/2
  V_0/1 -> Display/1, Subtract/1, Nominal liquid volume/1, Nominal gas volume/1
  Current volume (liq)/1 -> Sum/1, V_liq/1
  T_0/1 -> Gain Gain/3("T_0 "), Reference Density/1(T_Salt [k])
  [f_cv_0] -> Nominal gas volume/2
  Nominal gas volume/1 -> Gain Gain/1(Vol. Gas 0), Nominal liquid volume/2
  T/1 -> Gain Gain/2(T), Current Density/1(T_Salt [k])
  Sum/1 -> Subtract/2
  Gain Gain/1(V Gas) -> V_gas/1, Sum/2
  [V_R1_excess] -> Sum3/8
  [V_UH_excess] -> Sum3/4
  Subtract/1 -> Sum3/2
  [V_R2_excess] -> Sum3/7
  [V_LH_excess] -> Sum3/9
  [V_P101_excess] -> Sum3/1
  [V_P100_excess] -> Sum3/3
  [V_P102_excess] -> Sum3/11
  [V_HX_excess] -> Sum3/12
  [V_R4_excess] -> Sum3/5
  [V_CA_excess] -> Sum3/10
  [V_R3_excess] -> Sum3/6
  Sum3/1 -> FP Excess/1

== system Xe_Model_Redo_June_26/CONSTANTS/V FP1 ==
  note: Total Current Vol
  note: FS Volume W Thermal Expansion
  V_0 : Inport
  T_0 : Inport  Port=2
  T : Inport  Port=3
  Current Density : Subsystem
  Current volume (liq) : Product  Inputs=*/
  Display : Display
      settings: Format=short_e
  Gain : Gain  Gain=1.1
  Gain Gain : Subsystem
  Nominal Mass of Fuel Salt : Product
  Nominal gas volume : Product
  Nominal liquid volume : Sum  Inputs=+-
  Reference Density : Subsystem
  Subtract : Sum  Inputs=-+
  Sum : Sum
  Sum3 : Sum  Inputs=12
  V_liq : Outport
  FP Excess : Outport  Port=2
  V_gas : Outport  Port=3
  wires:
  Nominal Mass of Fuel Salt/1 -> Current volume (liq)/1
  Current Density/1(rho_FS [kg/m^3]) -> Current volume (liq)/2
  Nominal liquid volume/1 -> Nominal Mass of Fuel Salt/1
  Reference Density/1(rho_FS [kg/m^3]) -> Nominal Mass of Fuel Salt/2
  V_0/1 -> Display/1, Subtract/1, Nominal liquid volume/1, Nominal gas volume/1
  Current volume (liq)/1 -> Sum/1, V_liq/1
  T_0/1 -> Gain Gain/3("T_0 "), Reference Density/1(T_Salt [k])
  [f_cv_0] -> Nominal gas volume/2
  T/1 -> Gain/1
  Nominal gas volume/1 -> Gain Gain/1(Vol. Gas 0), Nominal liquid volume/2
  Gain/1 -> Gain Gain/2(T), Current Density/1(T_Salt [k])
  Sum/1 -> Subtract/2
  Gain Gain/1(V Gas) -> V_gas/1, Sum/2
  [V_R1_excess] -> Sum3/8
  [V_UH_excess] -> Sum3/4
  Subtract/1 -> Sum3/2
  [V_R2_excess] -> Sum3/7
  [V_LH_excess] -> Sum3/9
  [V_P101_excess] -> Sum3/1
  [V_P100_excess] -> Sum3/3
  [V_P102_excess] -> Sum3/11
  [V_HX_excess] -> Sum3/12
  [V_R4_excess] -> Sum3/5
  [V_CA_excess] -> Sum3/10
  [V_R3_excess] -> Sum3/6
  Sum3/1 -> FP Excess/1

== system Xe_Model_Redo_June_26/CONSTANTS/V HX ==
  note: Total Current Vol
  note: FS Volume W Thermal Expansion
  V_0 : Inport
  T_0 : Inport  Port=2
  T : Inport  Port=3
  Current Density : Subsystem
  Current volume (liq) : Product  Inputs=*/
  Display : Display
      settings: Format=short_e
  Gain Gain : Subsystem
  Nominal Mass of Fuel Salt : Product
  Nominal gas volume : Product
  Nominal liquid volume : Sum  Inputs=+-
  Reference Density : Subsystem
  Subtract : Sum  Inputs=-+
  Sum : Sum
  Sum1 : Sum  Inputs=+-
  V_liq : Outport
  V_excess_liq : Outport  Port=2
  V_gas : Outport  Port=3
  wires:
  Nominal Mass of Fuel Salt/1 -> Current volume (liq)/1
  Current Density/1(rho_FS [kg/m^3]) -> Current volume (liq)/2
  Nominal liquid volume/1 -> Nominal Mass of Fuel Salt/1
  Reference Density/1(rho_FS [kg/m^3]) -> Nominal Mass of Fuel Salt/2
  V_0/1 -> Display/1, Sum1/1, Subtract/1, Nominal liquid volume/1, Nominal gas volume/1
  Current volume (liq)/1 -> Sum/1
  T_0/1 -> Gain Gain/3("T_0 "), Reference Density/1(T_Salt [k])
  Subtract/1 -> V_excess_liq/1
  [f_cv_0] -> Nominal gas volume/2
  Nominal gas volume/1 -> Gain Gain/1(Vol. Gas 0), Nominal liquid volume/2
  T/1 -> Gain Gain/2(T), Current Density/1(T_Salt [k])
  Sum/1 -> Subtract/2
  Gain Gain/1(V Gas) -> V_gas/1, Sum1/2, Sum/2
  Sum1/1 -> V_liq/1

== system Xe_Model_Redo_June_26/CONSTANTS/V LH ==
  note: Total Current Vol
  note: FS Volume W Thermal Expansion
  V_0 : Inport
  T_0 : Inport  Port=2
  T : Inport  Port=3
  Current Density : Subsystem
  Current volume (liq) : Product  Inputs=*/
  Display : Display
      settings: Format=short_e
  Gain Gain : Subsystem
  Nominal Mass of Fuel Salt : Product
  Nominal gas volume : Product
  Nominal liquid volume : Sum  Inputs=+-
  Reference Density : Subsystem
  Subtract : Sum  Inputs=-+
  Sum : Sum
  Sum1 : Sum  Inputs=+-
  V_liq : Outport
  V_excess_liq : Outport  Port=2
  V_gas : Outport  Port=3
  wires:
  Nominal Mass of Fuel Salt/1 -> Current volume (liq)/1
  Current Density/1(rho_FS [kg/m^3]) -> Current volume (liq)/2
  Nominal liquid volume/1 -> Nominal Mass of Fuel Salt/1
  Reference Density/1(rho_FS [kg/m^3]) -> Nominal Mass of Fuel Salt/2
  V_0/1 -> Display/1, Sum1/1, Subtract/1, Nominal liquid volume/1, Nominal gas volume/1
  Current volume (liq)/1 -> Sum/1
  T_0/1 -> Gain Gain/3("T_0 "), Reference Density/1(T_Salt [k])
  Subtract/1 -> V_excess_liq/1
  [f_cv_0] -> Nominal gas volume/2
  Nominal gas volume/1 -> Gain Gain/1(Vol. Gas 0), Nominal liquid volume/2
  T/1 -> Gain Gain/2(T), Current Density/1(T_Salt [k])
  Sum/1 -> Subtract/2
  Gain Gain/1(V Gas) -> V_gas/1, Sum1/2, Sum/2
  Sum1/1 -> V_liq/1

== system Xe_Model_Redo_June_26/CONSTANTS/V P100 ==
  note: Total Current Vol
  note: FS Volume W Thermal Expansion
  V_0 : Inport
  T_0 : Inport  Port=2
  T : Inport  Port=3
  Current Density : Subsystem
  Current volume (liq) : Product  Inputs=*/
  Display : Display
      settings: Format=short_e
  Gain Gain : Subsystem
  Nominal Mass of Fuel Salt : Product
  Nominal gas volume : Product
  Nominal liquid volume : Sum  Inputs=+-
  Reference Density : Subsystem
  Subtract : Sum  Inputs=-+
  Sum : Sum
  Sum1 : Sum  Inputs=+-
  V_liq : Outport
  V_excess_liq : Outport  Port=2
  V_gas : Outport  Port=3
  wires:
  Nominal Mass of Fuel Salt/1 -> Current volume (liq)/1
  Current Density/1(rho_FS [kg/m^3]) -> Current volume (liq)/2
  Nominal liquid volume/1 -> Nominal Mass of Fuel Salt/1
  Reference Density/1(rho_FS [kg/m^3]) -> Nominal Mass of Fuel Salt/2
  V_0/1 -> Display/1, Sum1/1, Subtract/1, Nominal liquid volume/1, Nominal gas volume/1
  Current volume (liq)/1 -> Sum/1
  T_0/1 -> Gain Gain/3("T_0 "), Reference Density/1(T_Salt [k])
  Subtract/1 -> V_excess_liq/1
  [f_cv_0] -> Nominal gas volume/2
  Nominal gas volume/1 -> Gain Gain/1(Vol. Gas 0), Nominal liquid volume/2
  T/1 -> Gain Gain/2(T), Current Density/1(T_Salt [k])
  Sum/1 -> Subtract/2
  Gain Gain/1(V Gas) -> V_gas/1, Sum1/2, Sum/2
  Sum1/1 -> V_liq/1

== system Xe_Model_Redo_June_26/CONSTANTS/V P101 ==
  note: Total Current Vol
  note: FS Volume W Thermal Expansion
  V_0 : Inport
  T_0 : Inport  Port=2
  T : Inport  Port=3
  Current Density : Subsystem
  Current volume (liq) : Product  Inputs=*/
  Display : Display
      settings: Format=short_e
  Gain Gain : Subsystem
  Nominal Mass of Fuel Salt : Product
  Nominal gas volume : Product
  Nominal liquid volume : Sum  Inputs=+-
  Reference Density : Subsystem
  Subtract : Sum  Inputs=-+
  Sum : Sum
  Sum1 : Sum  Inputs=+-
  V_liq : Outport
  V_excess_liq : Outport  Port=2
  V_gas : Outport  Port=3
  wires:
  Nominal Mass of Fuel Salt/1 -> Current volume (liq)/1
  Current Density/1(rho_FS [kg/m^3]) -> Current volume (liq)/2
  Nominal liquid volume/1 -> Nominal Mass of Fuel Salt/1
  Reference Density/1(rho_FS [kg/m^3]) -> Nominal Mass of Fuel Salt/2
  V_0/1 -> Display/1, Sum1/1, Subtract/1, Nominal liquid volume/1, Nominal gas volume/1
  Current volume (liq)/1 -> Sum/1
  T_0/1 -> Gain Gain/3("T_0 "), Reference Density/1(T_Salt [k])
  Subtract/1 -> V_excess_liq/1
  [f_cv_0] -> Nominal gas volume/2
  Nominal gas volume/1 -> Gain Gain/1(Vol. Gas 0), Nominal liquid volume/2
  T/1 -> Gain Gain/2(T), Current Density/1(T_Salt [k])
  Sum/1 -> Subtract/2
  Gain Gain/1(V Gas) -> V_gas/1, Sum1/2, Sum/2
  Sum1/1 -> V_liq/1

== system Xe_Model_Redo_June_26/CONSTANTS/V P102 ==
  note: Total Current Vol
  note: FS Volume W Thermal Expansion
  V_0 : Inport
  T_0 : Inport  Port=2
  T : Inport  Port=3
  Current Density : Subsystem
  Current volume (liq) : Product  Inputs=*/
  Display : Display
      settings: Format=short_e
  Gain Gain : Subsystem
  Nominal Mass of Fuel Salt : Product
  Nominal gas volume : Product
  Nominal liquid volume : Sum  Inputs=+-
  Reference Density : Subsystem
  Subtract : Sum  Inputs=-+
  Sum : Sum
  Sum1 : Sum  Inputs=+-
  V_liq : Outport
  V_excess_liq : Outport  Port=2
  V_gas : Outport  Port=3
  wires:
  Nominal Mass of Fuel Salt/1 -> Current volume (liq)/1
  Current Density/1(rho_FS [kg/m^3]) -> Current volume (liq)/2
  Nominal liquid volume/1 -> Nominal Mass of Fuel Salt/1
  Reference Density/1(rho_FS [kg/m^3]) -> Nominal Mass of Fuel Salt/2
  V_0/1 -> Display/1, Sum1/1, Subtract/1, Nominal liquid volume/1, Nominal gas volume/1
  Current volume (liq)/1 -> Sum/1
  T_0/1 -> Gain Gain/3("T_0 "), Reference Density/1(T_Salt [k])
  Subtract/1 -> V_excess_liq/1
  [f_cv_0] -> Nominal gas volume/2
  Nominal gas volume/1 -> Gain Gain/1(Vol. Gas 0), Nominal liquid volume/2
  T/1 -> Gain Gain/2(T), Current Density/1(T_Salt [k])
  Sum/1 -> Subtract/2
  Gain Gain/1(V Gas) -> V_gas/1, Sum1/2, Sum/2
  Sum1/1 -> V_liq/1

== system Xe_Model_Redo_June_26/CONSTANTS/V R1 ==
  note: Total Current Vol
  note: FS Volume W Thermal Expansion
  V_0 : Inport
  T_0 : Inport  Port=2
  T : Inport  Port=3
  Current Density : Subsystem
  Current volume (liq) : Product  Inputs=*/
  Display : Display
      settings: Format=short_e
  Gain Gain : Subsystem
  Nominal Mass of Fuel Salt : Product
  Nominal gas volume : Product
  Nominal liquid volume : Sum  Inputs=+-
  Reference Density : Subsystem
  Subtract : Sum  Inputs=-+
  Sum : Sum
  Sum1 : Sum  Inputs=+-
  V_liq : Outport
  V_excess_liq : Outport  Port=2
  V_gas : Outport  Port=3
  wires:
  Nominal Mass of Fuel Salt/1 -> Current volume (liq)/1
  Current Density/1(rho_FS [kg/m^3]) -> Current volume (liq)/2
  Nominal liquid volume/1 -> Nominal Mass of Fuel Salt/1
  Reference Density/1(rho_FS [kg/m^3]) -> Nominal Mass of Fuel Salt/2
  V_0/1 -> Display/1, Sum1/1, Subtract/1, Nominal liquid volume/1, Nominal gas volume/1
  Current volume (liq)/1 -> Sum/1
  T_0/1 -> Gain Gain/3("T_0 "), Reference Density/1(T_Salt [k])
  Subtract/1 -> V_excess_liq/1
  [f_cv_0] -> Nominal gas volume/2
  Nominal gas volume/1 -> Gain Gain/1(Vol. Gas 0), Nominal liquid volume/2
  T/1 -> Gain Gain/2(T), Current Density/1(T_Salt [k])
  Sum/1 -> Subtract/2
  Gain Gain/1(V Gas) -> V_gas/1, Sum1/2, Sum/2
  Sum1/1 -> V_liq/1

== system Xe_Model_Redo_June_26/CONSTANTS/V R2 ==
  note: Total Current Vol
  note: FS Volume W Thermal Expansion
  V_0 : Inport
  T_0 : Inport  Port=2
  T : Inport  Port=3
  Current Density : Subsystem
  Current volume (liq) : Product  Inputs=*/
  Display : Display
      settings: Format=short_e
  Gain Gain : Subsystem
  Nominal Mass of Fuel Salt : Product
  Nominal gas volume : Product
  Nominal liquid volume : Sum  Inputs=+-
  Reference Density : Subsystem
  Subtract : Sum  Inputs=-+
  Sum : Sum
  Sum1 : Sum  Inputs=+-
  V_liq : Outport
  V_excess_liq : Outport  Port=2
  V_gas : Outport  Port=3
  wires:
  Nominal Mass of Fuel Salt/1 -> Current volume (liq)/1
  Current Density/1(rho_FS [kg/m^3]) -> Current volume (liq)/2
  Nominal liquid volume/1 -> Nominal Mass of Fuel Salt/1
  Reference Density/1(rho_FS [kg/m^3]) -> Nominal Mass of Fuel Salt/2
  V_0/1 -> Display/1, Sum1/1, Subtract/1, Nominal liquid volume/1, Nominal gas volume/1
  Current volume (liq)/1 -> Sum/1
  T_0/1 -> Gain Gain/3("T_0 "), Reference Density/1(T_Salt [k])
  Subtract/1 -> V_excess_liq/1
  [f_cv_0] -> Nominal gas volume/2
  Nominal gas volume/1 -> Gain Gain/1(Vol. Gas 0), Nominal liquid volume/2
  T/1 -> Gain Gain/2(T), Current Density/1(T_Salt [k])
  Sum/1 -> Subtract/2
  Gain Gain/1(V Gas) -> V_gas/1, Sum1/2, Sum/2
  Sum1/1 -> V_liq/1

== system Xe_Model_Redo_June_26/CONSTANTS/V R3 ==
  note: Total Current Vol
  note: FS Volume W Thermal Expansion
  V_0 : Inport
  T_0 : Inport  Port=2
  T : Inport  Port=3
  Current Density : Subsystem
  Current volume (liq) : Product  Inputs=*/
  Display : Display
      settings: Format=short_e
  Gain Gain : Subsystem
  Nominal Mass of Fuel Salt : Product
  Nominal gas volume : Product
  Nominal liquid volume : Sum  Inputs=+-
  Reference Density : Subsystem
  Subtract : Sum  Inputs=-+
  Sum : Sum
  Sum1 : Sum  Inputs=+-
  V_liq : Outport
  V_excess_liq : Outport  Port=2
  V_gas : Outport  Port=3
  wires:
  Nominal Mass of Fuel Salt/1 -> Current volume (liq)/1
  Current Density/1(rho_FS [kg/m^3]) -> Current volume (liq)/2
  Nominal liquid volume/1 -> Nominal Mass of Fuel Salt/1
  Reference Density/1(rho_FS [kg/m^3]) -> Nominal Mass of Fuel Salt/2
  V_0/1 -> Display/1, Sum1/1, Subtract/1, Nominal liquid volume/1, Nominal gas volume/1
  Current volume (liq)/1 -> Sum/1
  T_0/1 -> Gain Gain/3("T_0 "), Reference Density/1(T_Salt [k])
  Subtract/1 -> V_excess_liq/1
  [f_cv_0] -> Nominal gas volume/2
  Nominal gas volume/1 -> Gain Gain/1(Vol. Gas 0), Nominal liquid volume/2
  T/1 -> Gain Gain/2(T), Current Density/1(T_Salt [k])
  Sum/1 -> Subtract/2
  Gain Gain/1(V Gas) -> V_gas/1, Sum1/2, Sum/2
  Sum1/1 -> V_liq/1

== system Xe_Model_Redo_June_26/CONSTANTS/V R4 ==
  note: Total Current Vol
  note: FS Volume W Thermal Expansion
  V_0 : Inport
  T_0 : Inport  Port=2
  T : Inport  Port=3
  Current Density : Subsystem
  Current volume (liq) : Product  Inputs=*/
  Display : Display
      settings: Format=short_e
  Gain Gain : Subsystem
  Nominal Mass of Fuel Salt : Product
  Nominal gas volume : Product
  Nominal liquid volume : Sum  Inputs=+-
  Reference Density : Subsystem
  Subtract : Sum  Inputs=-+
  Sum : Sum
  Sum1 : Sum  Inputs=+-
  V_liq : Outport
  V_excess_liq : Outport  Port=2
  V_gas : Outport  Port=3
  wires:
  Nominal Mass of Fuel Salt/1 -> Current volume (liq)/1
  Current Density/1(rho_FS [kg/m^3]) -> Current volume (liq)/2
  Nominal liquid volume/1 -> Nominal Mass of Fuel Salt/1
  Reference Density/1(rho_FS [kg/m^3]) -> Nominal Mass of Fuel Salt/2
  V_0/1 -> Display/1, Sum1/1, Subtract/1, Nominal liquid volume/1, Nominal gas volume/1
  Current volume (liq)/1 -> Sum/1
  T_0/1 -> Gain Gain/3("T_0 "), Reference Density/1(T_Salt [k])
  Subtract/1 -> V_excess_liq/1
  [f_cv_0] -> Nominal gas volume/2
  Nominal gas volume/1 -> Gain Gain/1(Vol. Gas 0), Nominal liquid volume/2
  T/1 -> Gain Gain/2(T), Current Density/1(T_Salt [k])
  Sum/1 -> Subtract/2
  Gain Gain/1(V Gas) -> V_gas/1, Sum1/2, Sum/2
  Sum1/1 -> V_liq/1

== system Xe_Model_Redo_June_26/CONSTANTS/V UH ==
  note: Total Current Vol
  note: FS Volume W Thermal Expansion
  V_0 : Inport
  T_0 : Inport  Port=2
  T : Inport  Port=3
  Current Density : Subsystem
  Current volume (liq) : Product  Inputs=*/
  Display : Display
      settings: Format=short_e
  Gain Gain : Subsystem
  Nominal Mass of Fuel Salt : Product
  Nominal gas volume : Product
  Nominal liquid volume : Sum  Inputs=+-
  Reference Density : Subsystem
  Subtract : Sum  Inputs=-+
  Sum : Sum
  Sum1 : Sum  Inputs=+-
  V_liq : Outport
  V_excess_liq : Outport  Port=2
  V_gas : Outport  Port=3
  wires:
  Nominal Mass of Fuel Salt/1 -> Current volume (liq)/1
  Current Density/1(rho_FS [kg/m^3]) -> Current volume (liq)/2
  Nominal liquid volume/1 -> Nominal Mass of Fuel Salt/1
  Reference Density/1(rho_FS [kg/m^3]) -> Nominal Mass of Fuel Salt/2
  V_0/1 -> Display/1, Sum1/1, Subtract/1, Nominal liquid volume/1, Nominal gas volume/1
  Current volume (liq)/1 -> Sum/1
  T_0/1 -> Gain Gain/3("T_0 "), Reference Density/1(T_Salt [k])
  Subtract/1 -> V_excess_liq/1
  [f_cv_0] -> Nominal gas volume/2
  Nominal gas volume/1 -> Gain Gain/1(Vol. Gas 0), Nominal liquid volume/2
  T/1 -> Gain Gain/2(T), Current Density/1(T_Salt [k])
  Sum/1 -> Subtract/2
  Gain Gain/1(V Gas) -> V_gas/1, Sum1/2, Sum/2
  Sum1/1 -> V_liq/1

== system Xe_Model_Redo_June_26/Graphite /Graphite Region 1 ==
  N_Xe_FS : Inport
  Graphite MTC R1 : Subsystem
  Graphite Stringer : Subsystem
  Lumped Parameter Graphite Model : Subsystem
  Product : Product  Inputs=3
  Scope : Scope
  C_Xe_GS_Max : Outport
  C_Xe_GS_Mean : Outport  Port=2
  Nd_Xe_FS->GS : Outport  Port=3
  wires:
  [U_FC_R1] -> Graphite MTC R1/2(U_FC [m/s])
  [phi_G_R_1] -> Graphite Stringer/2(phi)
  Product/1 -> Nd_Xe_FS->GS/1
  [T_G_R_1] -> Graphite Stringer/1(T)
  Graphite Stringer/2(C_Xe_GS_Mean) -> Lumped Parameter Graphite Model/1(PDE), C_Xe_GS_Mean/1  "PDE"
  Graphite Stringer/3(J_Xe_FS->GS) -> Product/1
  Graphite Stringer/1(C_Xe_GS_Max) -> C_Xe_GS_Max/1
  [A_1_FC] -> Product/2
  [N_FC_R1] -> Product/3
  N_Xe_FS/1 -> Lumped Parameter Graphite Model/4(In4), Graphite Stringer/4(N_XE_FS)
  Graphite MTC R1/1(k_m_g [m/s]) -> Lumped Parameter Graphite Model/3(In3), Graphite Stringer/3(k_m_g)
  [T_G_R_1] -> Lumped Parameter Graphite Model/2(In2), Graphite MTC R1/1(T_Salt)
  Lumped Parameter Graphite Model/1(Out1) -> Scope/1

== system Xe_Model_Redo_June_26/Graphite /Graphite Region 2 ==
  N_Xe_FS : Inport
  Graphite MTC R1 : Subsystem
  Graphite Stringer : Subsystem
  Product : Product  Inputs=3
  C_Xe_GS_Max : Outport
  C_Xe_GS_Mean : Outport  Port=2
  Nd_Xe_FS->GS : Outport  Port=3
  wires:
  [U_FC_R2] -> Graphite MTC R1/2(U_FC [m/s])
  [phi_G_R_2] -> Graphite Stringer/2(phi)
  [T_G_R_2] -> Graphite MTC R1/1(T_Salt)
  Product/1 -> Nd_Xe_FS->GS/1
  [T_G_R_2] -> Graphite Stringer/1(T)
  N_Xe_FS/1 -> Graphite Stringer/4(N_XE_FS)
  Graphite Stringer/2(C_Xe_GS_Mean) -> C_Xe_GS_Mean/1
  Graphite Stringer/3(J_Xe_FS->GS) -> Product/1
  Graphite Stringer/1(C_Xe_GS_Max) -> C_Xe_GS_Max/1
  [A_1_FC] -> Product/2
  [N_FC_R2] -> Product/3
  Graphite MTC R1/1(k_m_g [m/s]) -> Graphite Stringer/3(k_m_g)
